simulink model "double_dm2"  (R2023a)
settings: Solver=VariableStepAuto  StartTime=0.0  StopTime=10.0  RelTol=1e-3
settings Model: Creator=isaac  LastModifiedBy=isaac

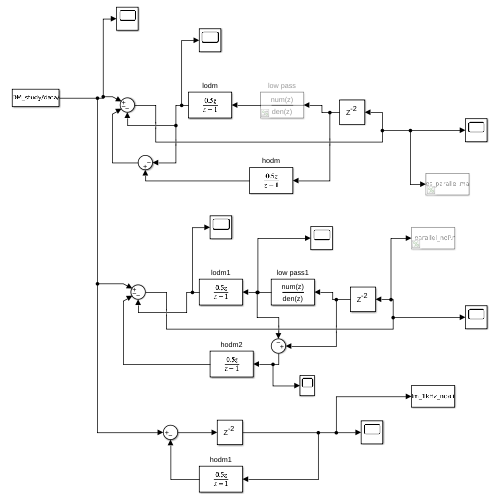
[thumbnail: Simulink's stored preview of the top-level diagram]
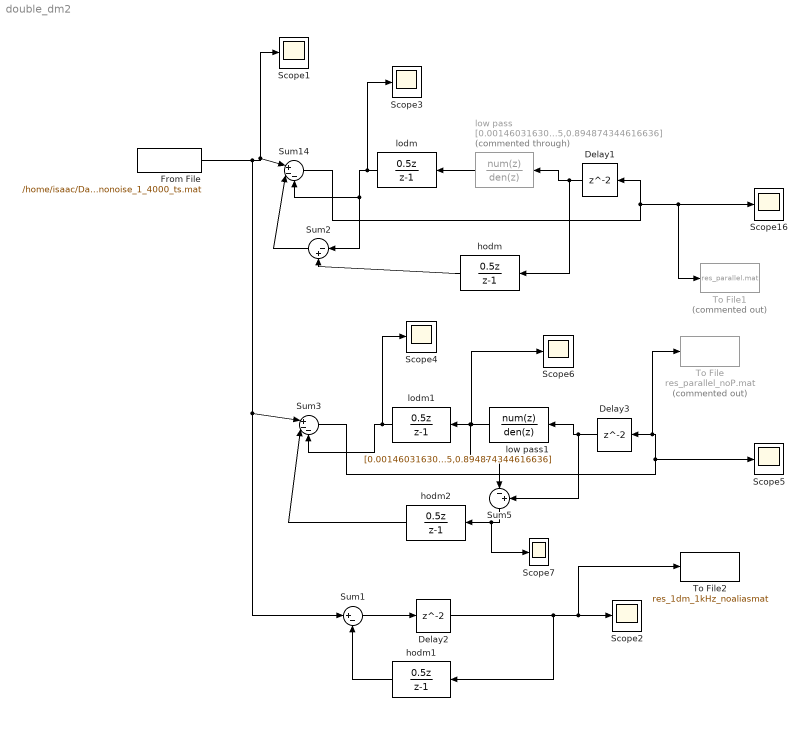
== system double_dm2 ==
  Delay1 : Delay  SampleTime=1/4000
  Delay2 : Delay  SampleTime=1/1000
  Delay3 : Delay  SampleTime=1/4000
  From File : FromFile  FileName=/home/isaac/Data-Driven-Control-for-AO/2DM_study/data/single_mode_dist_nonoise_1_4000_ts.mat  SampleTime=1/4000
  Scope{1..7,16} (8 alike) : Scope
  Sum1 : Sum  Inputs=|+-
  Sum14 : Sum  Inputs=|+--
  Sum2 : Sum  Inputs=|-+
  Sum3 : Sum  Inputs=|+--
  Sum5 : Sum  Inputs=|-+
  To File : ToFile  Commented=on  Filename=res_parallel_noP.mat  MatrixName=data  SampleTime=1/4000
  To File1 : ToFile  Commented=on  Filename=res_parallel.mat  MatrixName=data  SampleTime=1/4000
  To File2 : ToFile  Filename=res_1dm_1kHz_noaliasmat  MatrixName=data  SampleTime=1/4000
  hodm : DiscreteTransferFcn  Numerator=[0.5 0]  Denominator=[1 -1]  SampleTime=1/4000
  hodm1 : DiscreteTransferFcn  Numerator=[0.5 0]  Denominator=[1 -1]  SampleTime=1/1000
  hodm2 : DiscreteTransferFcn  Numerator=[0.5 0]  Denominator=[1 -1]  SampleTime=1/4000
  lodm : DiscreteTransferFcn  Numerator=[0.5 0]  Denominator=[1 -1]  SampleTime=0.001
  lodm1 : DiscreteTransferFcn  Numerator=[0.5 0]  Denominator=[1 -1]  SampleTime=0.001
  low pass : DiscreteFilter  Commented=through  Numerator=[0.001460316305528,0.002920632611055,0.001460316305528]  Denominator=[1,-1.889033079394525,0.894874344616636]  SampleTime=1/4000
  low pass1 : DiscreteFilter  Numerator=[0.001460316305528,0.002920632611055,0.001460316305528]  Denominator=[1,-1.889033079394525,0.894874344616636]  SampleTime=1/4000
  wires:
  lodm/1 -> Scope3/1, Sum14/3, Sum2/1
  Sum1/1 -> Delay2/1
  From File/1 -> Sum3/1, Sum1/1, Scope1/1, Sum14/1
  Delay2/1 -> hodm1/1, To File2/1, Scope2/1
  Delay1/1 -> hodm/1, low pass/1
  low pass/1 -> lodm/1
  hodm1/1 -> Sum1/2
  hodm/1 -> Sum2/2
  Sum2/1 -> Sum14/2
  Sum14/1 -> To File1/1, Scope16/1, Delay1/1
  lodm1/1 -> Scope4/1, Sum3/3
  Delay3/1 -> Sum5/2, low pass1/1
  low pass1/1 -> Sum5/1, lodm1/1, Scope6/1
  Sum3/1 -> Scope5/1, To File/1, Delay3/1
  Sum5/1 -> hodm2/1, Scope7/1
  hodm2/1 -> Sum3/2
